simulink model "untitled"  (R2023b)
settings: Solver=VariableStepAuto  StartTime=0.0  StopTime=10  RelTol=1e-3
values from neighbouring files (symbols this model uses):
  A = [0, 1; -3, -4]    [e01.m]
  alpha = 1/[-(C-D*K)*inv(A-B*K)*B+D]    [e01.m]
  B = [0; 1]    [e01.m]
  C = [2 , 1]    [e01.m]
  D = 0    [e01.m]
  K = place(A, B, pk)    [e01.m]
  L = place(A', C', pl)'    [e01.m]
settings Model: Creator=Marco  LastModifiedBy=Marco

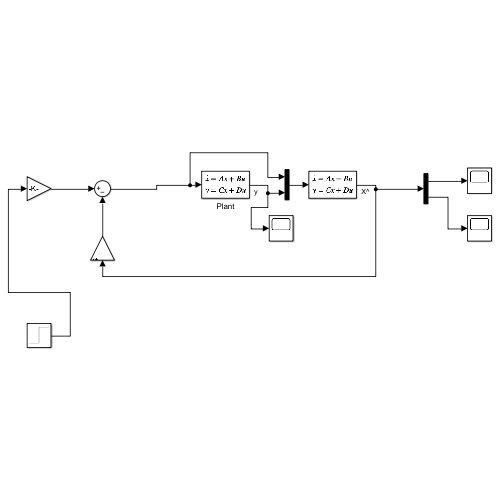
[thumbnail: Simulink's stored preview of the top-level diagram]
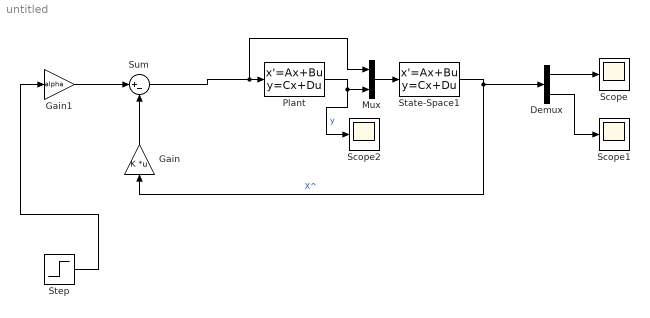
== system untitled ==
  Demux : Demux  Outputs=2
  Gain : Gain  Gain=K  Multiplication=Matrix(K*u) (u vector)
  Gain1 : Gain  Gain=alpha
  Mux : Mux  Inputs=2
  Plant : StateSpace  A=A  B=B  C=C  D=D  InitialCondition=0
  Scope : Scope
  Scope1 : Scope
  Scope2 : Scope
  State-Space1 : StateSpace  A=A-L*C  B=[B, L]  C=eye(2)  D=[0,0;0,0]  InitialCondition=0  ParameterTunability=Unconstrained  AllowTunableDMatrix=on
  Step : Step  Time=0  SampleTime=0
  Sum : Sum  Inputs=|+-
  wires:
  Mux/1 -> State-Space1/1
  Gain/1 -> Sum/2
  Gain1/1 -> Sum/1
  Step/1 -> Gain1/1
  State-Space1/1 -> Demux/1, Gain/1  "X^"
  Sum/1 -> Mux/1, Plant/1
  Plant/1 -> Scope2/1, Mux/2  "y"
  Demux/1 -> Scope/1
  Demux/2 -> Scope1/1
